simulink model "NavigationObserver_4"  (Simulink 8.3)
settings: configuration reference "mpc555rt_ref_debug_config" (kept outside this file)
values from neighbouring files (symbols this model uses):
  dt = 0.0192307692308    [newvars_4_25.mat]
  g = 32.174    [newvars_4_25.mat]
  P0_est_nav = [100 0 0 0 0 0 0 100 0 0 0 0 ... (36 elements, 6x6)]    [newvars_4_25.mat]
  Q_obs_nav = [0.001 0 0 0 0 0 0 0.001 0 0 0 0 ... (36 elements, 6x6)]    [newvars_4_25.mat]
  R_obs_nav = [0.001 0 0 0 0 0 0 0.001 0 0 0 0 ... (36 elements, 6x6)]    [newvars_4_25.mat]
  x0_est_nav = [0 0 200 0 0 0]    [newvars_4_25.mat]
libraries: simulink x1
(part 2 of 2)

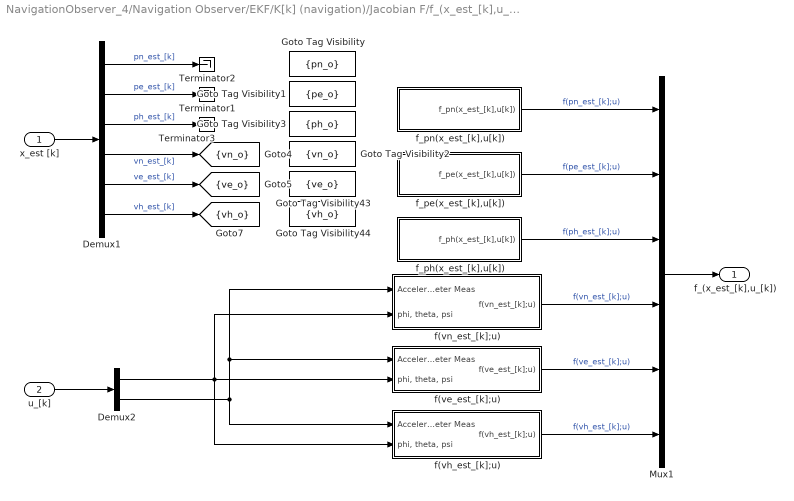
== system NavigationObserver_4/Navigation Observer/EKF/K[k] (navigation)/Jacobian F/f_(x_est_[k],u_[k])+delta_ve/f(x_est_[k],u_[k]) ==
  x_est [k] : Inport
  u_[k] : Inport  Port=2
  Demux1 : Demux  Outputs=6
  Demux2 : Demux  Outputs=2
  Goto Tag Visibility : GotoTagVisibility  GotoTag=pn_o
  Goto Tag Visibility1 : GotoTagVisibility  GotoTag=pe_o
  Goto Tag Visibility2 : GotoTagVisibility  GotoTag=vn_o
  Goto Tag Visibility3 : GotoTagVisibility  GotoTag=ph_o
  Goto Tag Visibility43 : GotoTagVisibility  GotoTag=ve_o
  Goto Tag Visibility44 : GotoTagVisibility  GotoTag=vh_o
  Mux1 : Mux  Inputs=6
  Terminator1 : Terminator
  Terminator2 : Terminator
  Terminator3 : Terminator
  f(ve_est_[k];u) : Subsystem
  f(vh_est_[k];u) : Subsystem
  f(vn_est_[k];u) : Subsystem
  f_pe(x_est_[k],u[k]) : Subsystem
  f_ph(x_est_[k],u[k]) : Subsystem
  f_pn(x_est_[k],u[k]) : Subsystem
  f_(x_est_[k],u_[k]) : Outport
  tag scope: ve_o=scoped, vh_o=scoped, vn_o=scoped
  wires:
  Demux2/2 -> f(vh_est_[k];u)/1(Accelerometer Meas), f(ve_est_[k];u)/1(Accelerometer Meas), f(vn_est_[k];u)/1(Accelerometer Meas)
  Demux2/1 -> f(vn_est_[k];u)/2("phi, theta, psi"), f(vh_est_[k];u)/2("phi, theta, psi"), f(ve_est_[k];u)/2("phi, theta, psi")
  u_[k]/1 -> Demux2/1
  f_pe(x_est_[k],u[k])/1(f_pe(x_est_[k],u[k])) -> Mux1/2  "f(pe_est_[k];u)"
  f_pn(x_est_[k],u[k])/1(f_pn(x_est_[k],u[k])) -> Mux1/1  "f(pn_est_[k];u)"
  f_ph(x_est_[k],u[k])/1(f_ph(x_est_[k],u[k])) -> Mux1/3  "f(ph_est_[k];u)"
  f(vn_est_[k];u)/1(f(vn_est_[k];u)) -> Mux1/4  "f(vn_est_[k];u)"
  f(ve_est_[k];u)/1(f(ve_est_[k];u)) -> Mux1/5  "f(ve_est_[k];u)"
  Mux1/1 -> f_(x_est_[k],u_[k])/1
  f(vh_est_[k];u)/1(f(vh_est_[k];u)) -> Mux1/6  "f(vh_est_[k];u)"
  Demux1/5 -> [ve_o]  "ve_est_[k]"
  x_est [k]/1 -> Demux1/1
  Demux1/6 -> [vh_o]  "vh_est_[k]"
  Demux1/4 -> [vn_o]  "vn_est_[k]"
  Demux1/3 -> Terminator3/1  "ph_est_[k]"
  Demux1/2 -> Terminator1/1  "pe_est_[k]"
  Demux1/1 -> Terminator2/1  "pn_est_[k]"

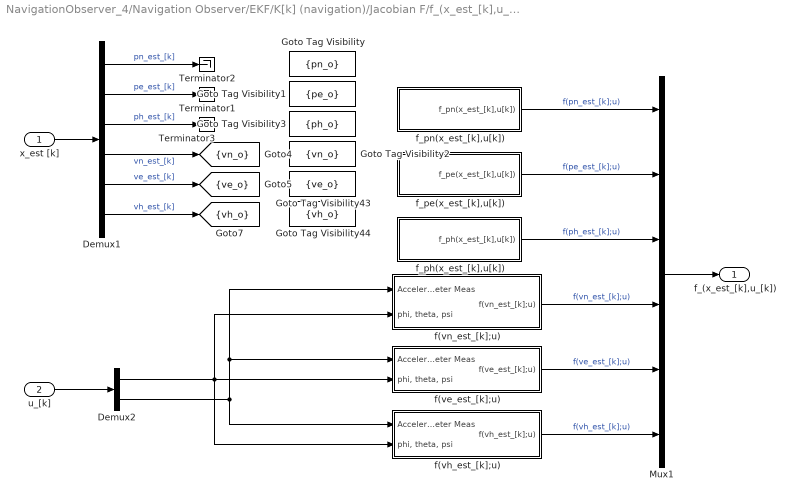
== system NavigationObserver_4/Navigation Observer/EKF/K[k] (navigation)/Jacobian F/f_(x_est_[k],u_[k])+delta_vh/f(x_est_[k],u_[k]) ==
  x_est [k] : Inport
  u_[k] : Inport  Port=2
  Demux1 : Demux  Outputs=6
  Demux2 : Demux  Outputs=2
  Goto Tag Visibility : GotoTagVisibility  GotoTag=pn_o
  Goto Tag Visibility1 : GotoTagVisibility  GotoTag=pe_o
  Goto Tag Visibility2 : GotoTagVisibility  GotoTag=vn_o
  Goto Tag Visibility3 : GotoTagVisibility  GotoTag=ph_o
  Goto Tag Visibility43 : GotoTagVisibility  GotoTag=ve_o
  Goto Tag Visibility44 : GotoTagVisibility  GotoTag=vh_o
  Mux1 : Mux  Inputs=6
  Terminator1 : Terminator
  Terminator2 : Terminator
  Terminator3 : Terminator
  f(ve_est_[k];u) : Subsystem
  f(vh_est_[k];u) : Subsystem
  f(vn_est_[k];u) : Subsystem
  f_pe(x_est_[k],u[k]) : Subsystem
  f_ph(x_est_[k],u[k]) : Subsystem
  f_pn(x_est_[k],u[k]) : Subsystem
  f_(x_est_[k],u_[k]) : Outport
  tag scope: ve_o=scoped, vh_o=scoped, vn_o=scoped
  wires:
  Demux2/2 -> f(vh_est_[k];u)/1(Accelerometer Meas), f(ve_est_[k];u)/1(Accelerometer Meas), f(vn_est_[k];u)/1(Accelerometer Meas)
  Demux2/1 -> f(vn_est_[k];u)/2("phi, theta, psi"), f(vh_est_[k];u)/2("phi, theta, psi"), f(ve_est_[k];u)/2("phi, theta, psi")
  u_[k]/1 -> Demux2/1
  f_pe(x_est_[k],u[k])/1(f_pe(x_est_[k],u[k])) -> Mux1/2  "f(pe_est_[k];u)"
  f_pn(x_est_[k],u[k])/1(f_pn(x_est_[k],u[k])) -> Mux1/1  "f(pn_est_[k];u)"
  f_ph(x_est_[k],u[k])/1(f_ph(x_est_[k],u[k])) -> Mux1/3  "f(ph_est_[k];u)"
  f(vn_est_[k];u)/1(f(vn_est_[k];u)) -> Mux1/4  "f(vn_est_[k];u)"
  f(ve_est_[k];u)/1(f(ve_est_[k];u)) -> Mux1/5  "f(ve_est_[k];u)"
  Mux1/1 -> f_(x_est_[k],u_[k])/1
  f(vh_est_[k];u)/1(f(vh_est_[k];u)) -> Mux1/6  "f(vh_est_[k];u)"
  Demux1/5 -> [ve_o]  "ve_est_[k]"
  x_est [k]/1 -> Demux1/1
  Demux1/6 -> [vh_o]  "vh_est_[k]"
  Demux1/4 -> [vn_o]  "vn_est_[k]"
  Demux1/3 -> Terminator3/1  "ph_est_[k]"
  Demux1/2 -> Terminator1/1  "pe_est_[k]"
  Demux1/1 -> Terminator2/1  "pn_est_[k]"

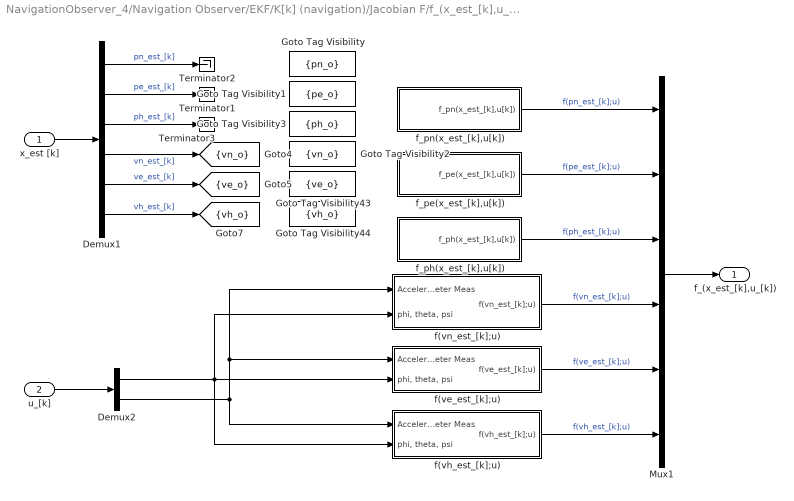
== system NavigationObserver_4/Navigation Observer/EKF/K[k] (navigation)/Jacobian F/f_(x_est_[k],u_[k])+delta_vn/f(x_est_[k],u_[k]) ==
  x_est [k] : Inport
  u_[k] : Inport  Port=2
  Demux1 : Demux  Outputs=6
  Demux2 : Demux  Outputs=2
  Goto Tag Visibility : GotoTagVisibility  GotoTag=pn_o
  Goto Tag Visibility1 : GotoTagVisibility  GotoTag=pe_o
  Goto Tag Visibility2 : GotoTagVisibility  GotoTag=vn_o
  Goto Tag Visibility3 : GotoTagVisibility  GotoTag=ph_o
  Goto Tag Visibility43 : GotoTagVisibility  GotoTag=ve_o
  Goto Tag Visibility44 : GotoTagVisibility  GotoTag=vh_o
  Mux1 : Mux  Inputs=6
  Terminator1 : Terminator
  Terminator2 : Terminator
  Terminator3 : Terminator
  f(ve_est_[k];u) : Subsystem
  f(vh_est_[k];u) : Subsystem
  f(vn_est_[k];u) : Subsystem
  f_pe(x_est_[k],u[k]) : Subsystem
  f_ph(x_est_[k],u[k]) : Subsystem
  f_pn(x_est_[k],u[k]) : Subsystem
  f_(x_est_[k],u_[k]) : Outport
  tag scope: ve_o=scoped, vh_o=scoped, vn_o=scoped
  wires:
  Demux2/2 -> f(vh_est_[k];u)/1(Accelerometer Meas), f(ve_est_[k];u)/1(Accelerometer Meas), f(vn_est_[k];u)/1(Accelerometer Meas)
  Demux2/1 -> f(vn_est_[k];u)/2("phi, theta, psi"), f(vh_est_[k];u)/2("phi, theta, psi"), f(ve_est_[k];u)/2("phi, theta, psi")
  u_[k]/1 -> Demux2/1
  f_pe(x_est_[k],u[k])/1(f_pe(x_est_[k],u[k])) -> Mux1/2  "f(pe_est_[k];u)"
  f_pn(x_est_[k],u[k])/1(f_pn(x_est_[k],u[k])) -> Mux1/1  "f(pn_est_[k];u)"
  f_ph(x_est_[k],u[k])/1(f_ph(x_est_[k],u[k])) -> Mux1/3  "f(ph_est_[k];u)"
  f(vn_est_[k];u)/1(f(vn_est_[k];u)) -> Mux1/4  "f(vn_est_[k];u)"
  f(ve_est_[k];u)/1(f(ve_est_[k];u)) -> Mux1/5  "f(ve_est_[k];u)"
  Mux1/1 -> f_(x_est_[k],u_[k])/1
  f(vh_est_[k];u)/1(f(vh_est_[k];u)) -> Mux1/6  "f(vh_est_[k];u)"
  Demux1/5 -> [ve_o]  "ve_est_[k]"
  x_est [k]/1 -> Demux1/1
  Demux1/6 -> [vh_o]  "vh_est_[k]"
  Demux1/4 -> [vn_o]  "vn_est_[k]"
  Demux1/3 -> Terminator3/1  "ph_est_[k]"
  Demux1/2 -> Terminator1/1  "pe_est_[k]"
  Demux1/1 -> Terminator2/1  "pn_est_[k]"

== system NavigationObserver_4/Navigation Observer/EKF/K[k] (navigation)/Jacobian F/f_(x_est_[k],u_[k])/f(x_est_[k],u_[k])/f(ve_est_[k];u) ==
  note: psi [rad]
  note: phi [rad]
  note: theta [rad]
  note: az [ft/sec2]
  note: ay [ft/sec2]
  note: ax [ft/sec2]
  Accelerometer Meas : Inport
  "phi, theta, psi" : Inport  Port=2
  Add1 : Sum
  Add2 : Sum  Inputs=+++
  Add3 : Sum  Inputs=-+
  Demux1 : Demux  Outputs=3
  Demux2 : Demux  Outputs=3
  Divide{1,4,6..7} (4 alike) : Product  Inputs=**
  Divide2 : Product  Inputs=***
  Divide3 : Product  Inputs=***
  Divide5 : Product  Inputs=***
  Trigonometric Function : Trigonometry
  Trigonometric Function1 : Trigonometry  Operator=cos
  Trigonometric Function2 : Trigonometry
  Trigonometric Function3 : Trigonometry
  Trigonometric Function4 : Trigonometry  Operator=cos
  Trigonometric Function5 : Trigonometry  Operator=cos
  f(ve_est_[k];u) : Outport
  wires:
  "phi, theta, psi"/1 -> Demux2/1
  Accelerometer Meas/1 -> Demux1/1
  Add2/1 -> f(ve_est_[k];u)/1
  Demux1/1 -> Divide3/1
  Trigonometric Function1/1 -> Divide3/2
  Add1/1 -> Divide1/1
  Divide4/1 -> Add1/1
  Divide2/1 -> Add1/2
  Divide3/1 -> Add2/1
  Divide1/1 -> Add2/2
  Divide6/1 -> Add3/1
  Divide5/1 -> Add3/2
  Add3/1 -> Divide7/1
  Divide7/1 -> Add2/3
  Trigonometric Function3/1 -> Divide2/3, Divide5/3, Divide3/3
  Trigonometric Function5/1 -> Divide4/1, Divide5/2
  Trigonometric Function4/1 -> Divide4/2, Divide6/2
  Trigonometric Function2/1 -> Divide2/1, Divide5/1
  Trigonometric Function/1 -> Divide2/2, Divide6/1
  Demux1/3 -> Divide7/2
  Demux1/2 -> Divide1/2
  Demux2/1 -> Trigonometric Function5/1, Trigonometric Function/1
  Demux2/2 -> Trigonometric Function1/1, Trigonometric Function2/1
  Demux2/3 -> Trigonometric Function4/1, Trigonometric Function3/1

== system NavigationObserver_4/Navigation Observer/EKF/K[k] (navigation)/Jacobian F/f_(x_est_[k],u_[k])/f(x_est_[k],u_[k])/f(vh_est_[k];u) ==
  note: phi [rad]
  note: theta [rad]
  note: az [ft/sec2]
  note: ay [ft/sec2]
  note: ax [ft/sec2]
  Accelerometer Meas : Inport
  "phi, theta, psi" : Inport  Port=2
  Add1 : Sum  Inputs=+--
  Demux1 : Demux  Outputs=3
  Demux2 : Demux  Outputs=3
  Divide1 : Product  Inputs=***
  Divide2 : Product  Inputs=**
  Divide3 : Product  Inputs=***
  Sum : Sum  Inputs=|+-  SampleTime=dt
  Terminator2 : Terminator
  Trigonometric Function : Trigonometry
  Trigonometric Function1 : Trigonometry  Operator=cos
  Trigonometric Function2 : Trigonometry
  Trigonometric Function4 : Trigonometry  Operator=cos
  Trigonometric Function5 : Trigonometry  Operator=cos
  gravity : Constant  Value=g
  f(vh_est_[k];u) : Outport
  wires:
  gravity/1 -> Sum/2
  Sum/1 -> f(vh_est_[k];u)/1
  Add1/1 -> Sum/1
  Demux2/3 -> Terminator2/1
  "phi, theta, psi"/1 -> Demux2/1
  Accelerometer Meas/1 -> Demux1/1
  Demux1/1 -> Divide2/1
  Trigonometric Function/1 -> Divide2/2
  Trigonometric Function1/1 -> Divide3/1
  Trigonometric Function2/1 -> Divide3/2
  Demux1/2 -> Divide3/3
  Divide3/1 -> Add1/2
  Divide2/1 -> Add1/1
  Trigonometric Function4/1 -> Divide1/1
  Trigonometric Function5/1 -> Divide1/2
  Demux1/3 -> Divide1/3
  Divide1/1 -> Add1/3
  Demux2/2 -> Trigonometric Function/1, Trigonometric Function1/1, Trigonometric Function5/1
  Demux2/1 -> Trigonometric Function2/1, Trigonometric Function4/1

== system NavigationObserver_4/Navigation Observer/EKF/K[k] (navigation)/Jacobian F/f_(x_est_[k],u_[k])/f(x_est_[k],u_[k])/f(vn_est_[k];u) ==
  note: psi [rad]
  note: phi [rad]
  note: theta [rad]
  note: az [ft/sec2]
  note: ay [ft/sec2]
  note: ax [ft/sec2]
  Accelerometer Meas : Inport
  "phi, theta, psi" : Inport  Port=2
  Add1 : Sum  Inputs=-+
  Add2 : Sum  Inputs=+++
  Add3 : Sum
  Demux1 : Demux  Outputs=3
  Demux2 : Demux  Outputs=3
  Divide{1,4,6..7} (4 alike) : Product  Inputs=**
  Divide2 : Product  Inputs=***
  Divide3 : Product  Inputs=***
  Divide5 : Product  Inputs=***
  Trigonometric Function : Trigonometry
  Trigonometric Function1 : Trigonometry  Operator=cos
  Trigonometric Function2 : Trigonometry
  Trigonometric Function3 : Trigonometry
  Trigonometric Function4 : Trigonometry  Operator=cos
  Trigonometric Function5 : Trigonometry  Operator=cos
  f(vn_est_[k];u) : Outport
  wires:
  Accelerometer Meas/1 -> Demux1/1
  Demux1/1 -> Divide3/1
  Demux1/2 -> Divide1/2
  Demux1/3 -> Divide7/2
  Add2/1 -> f(vn_est_[k];u)/1
  Demux2/2 -> Trigonometric Function1/1, Trigonometric Function2/1
  Demux2/1 -> Trigonometric Function5/1, Trigonometric Function/1
  Demux2/3 -> Trigonometric Function4/1, Trigonometric Function3/1
  Trigonometric Function1/1 -> Divide3/2
  Trigonometric Function4/1 -> Divide3/3, Divide2/3, Divide5/3
  Add1/1 -> Divide1/1
  Divide4/1 -> Add1/1
  Divide2/1 -> Add1/2
  Trigonometric Function5/1 -> Divide4/1, Divide5/2
  Trigonometric Function3/1 -> Divide4/2, Divide6/2
  Trigonometric Function2/1 -> Divide2/1, Divide5/1
  Trigonometric Function/1 -> Divide2/2, Divide6/1
  Divide3/1 -> Add2/1
  Divide1/1 -> Add2/2
  Divide6/1 -> Add3/1
  Divide5/1 -> Add3/2
  Add3/1 -> Divide7/1
  Divide7/1 -> Add2/3
  "phi, theta, psi"/1 -> Demux2/1

== system NavigationObserver_4/Navigation Observer/EKF/K[k] (navigation)/Jacobian F/f_(x_est_[k],u_[k])/f(x_est_[k],u_[k])/f_pe(x_est_[k],u[k]) ==
  Gain : Gain
  f_pe(x_est_[k],u[k]) : Outport
  wires:
  Gain/1 -> f_pe(x_est_[k],u[k])/1
  [ve_o] -> Gain/1

== system NavigationObserver_4/Navigation Observer/EKF/K[k] (navigation)/Jacobian F/f_(x_est_[k],u_[k])/f(x_est_[k],u_[k])/f_ph(x_est_[k],u[k]) ==
  Gain : Gain
  f_ph(x_est_[k],u[k]) : Outport
  wires:
  Gain/1 -> f_ph(x_est_[k],u[k])/1
  [vh_o] -> Gain/1

== system NavigationObserver_4/Navigation Observer/EKF/K[k] (navigation)/Jacobian F/f_(x_est_[k],u_[k])/f(x_est_[k],u_[k])/f_pn(x_est_[k],u[k]) ==
  Gain : Gain
  f_pn(x_est_[k],u[k]) : Outport
  wires:
  Gain/1 -> f_pn(x_est_[k],u[k])/1
  [vn_o] -> Gain/1

== system NavigationObserver_4/Navigation Observer/EKF/K[k] (navigation)/Jacobian F/f_(x_est_[k],u_[k])+delta_pe/f(x_est_[k],u_[k])/f(ve_est_[k];u) ==
  note: psi [rad]
  note: phi [rad]
  note: theta [rad]
  note: az [ft/sec2]
  note: ay [ft/sec2]
  note: ax [ft/sec2]
  Accelerometer Meas : Inport
  "phi, theta, psi" : Inport  Port=2
  Add1 : Sum
  Add2 : Sum  Inputs=+++
  Add3 : Sum  Inputs=-+
  Demux1 : Demux  Outputs=3
  Demux2 : Demux  Outputs=3
  Divide{1,4,6..7} (4 alike) : Product  Inputs=**
  Divide2 : Product  Inputs=***
  Divide3 : Product  Inputs=***
  Divide5 : Product  Inputs=***
  Trigonometric Function : Trigonometry
  Trigonometric Function1 : Trigonometry  Operator=cos
  Trigonometric Function2 : Trigonometry
  Trigonometric Function3 : Trigonometry
  Trigonometric Function4 : Trigonometry  Operator=cos
  Trigonometric Function5 : Trigonometry  Operator=cos
  f(ve_est_[k];u) : Outport
  wires:
  "phi, theta, psi"/1 -> Demux2/1
  Accelerometer Meas/1 -> Demux1/1
  Add2/1 -> f(ve_est_[k];u)/1
  Demux1/1 -> Divide3/1
  Trigonometric Function1/1 -> Divide3/2
  Add1/1 -> Divide1/1
  Divide4/1 -> Add1/1
  Divide2/1 -> Add1/2
  Divide3/1 -> Add2/1
  Divide1/1 -> Add2/2
  Divide6/1 -> Add3/1
  Divide5/1 -> Add3/2
  Add3/1 -> Divide7/1
  Divide7/1 -> Add2/3
  Trigonometric Function3/1 -> Divide2/3, Divide5/3, Divide3/3
  Trigonometric Function5/1 -> Divide4/1, Divide5/2
  Trigonometric Function4/1 -> Divide4/2, Divide6/2
  Trigonometric Function2/1 -> Divide2/1, Divide5/1
  Trigonometric Function/1 -> Divide2/2, Divide6/1
  Demux1/3 -> Divide7/2
  Demux1/2 -> Divide1/2
  Demux2/1 -> Trigonometric Function5/1, Trigonometric Function/1
  Demux2/2 -> Trigonometric Function1/1, Trigonometric Function2/1
  Demux2/3 -> Trigonometric Function4/1, Trigonometric Function3/1

== system NavigationObserver_4/Navigation Observer/EKF/K[k] (navigation)/Jacobian F/f_(x_est_[k],u_[k])+delta_pe/f(x_est_[k],u_[k])/f(vh_est_[k];u) ==
  note: phi [rad]
  note: theta [rad]
  note: az [ft/sec2]
  note: ay [ft/sec2]
  note: ax [ft/sec2]
  Accelerometer Meas : Inport
  "phi, theta, psi" : Inport  Port=2
  Add1 : Sum  Inputs=+--
  Demux1 : Demux  Outputs=3
  Demux2 : Demux  Outputs=3
  Divide1 : Product  Inputs=***
  Divide2 : Product  Inputs=**
  Divide3 : Product  Inputs=***
  Sum : Sum  Inputs=|+-  SampleTime=dt
  Terminator2 : Terminator
  Trigonometric Function : Trigonometry
  Trigonometric Function1 : Trigonometry  Operator=cos
  Trigonometric Function2 : Trigonometry
  Trigonometric Function4 : Trigonometry  Operator=cos
  Trigonometric Function5 : Trigonometry  Operator=cos
  gravity : Constant  Value=g
  f(vh_est_[k];u) : Outport
  wires:
  gravity/1 -> Sum/2
  Sum/1 -> f(vh_est_[k];u)/1
  Add1/1 -> Sum/1
  Demux2/3 -> Terminator2/1
  "phi, theta, psi"/1 -> Demux2/1
  Accelerometer Meas/1 -> Demux1/1
  Demux1/1 -> Divide2/1
  Trigonometric Function/1 -> Divide2/2
  Trigonometric Function1/1 -> Divide3/1
  Trigonometric Function2/1 -> Divide3/2
  Demux1/2 -> Divide3/3
  Divide3/1 -> Add1/2
  Divide2/1 -> Add1/1
  Trigonometric Function4/1 -> Divide1/1
  Trigonometric Function5/1 -> Divide1/2
  Demux1/3 -> Divide1/3
  Divide1/1 -> Add1/3
  Demux2/2 -> Trigonometric Function/1, Trigonometric Function1/1, Trigonometric Function5/1
  Demux2/1 -> Trigonometric Function2/1, Trigonometric Function4/1

== system NavigationObserver_4/Navigation Observer/EKF/K[k] (navigation)/Jacobian F/f_(x_est_[k],u_[k])+delta_pe/f(x_est_[k],u_[k])/f(vn_est_[k];u) ==
  note: psi [rad]
  note: phi [rad]
  note: theta [rad]
  note: az [ft/sec2]
  note: ay [ft/sec2]
  note: ax [ft/sec2]
  Accelerometer Meas : Inport
  "phi, theta, psi" : Inport  Port=2
  Add1 : Sum  Inputs=-+
  Add2 : Sum  Inputs=+++
  Add3 : Sum
  Demux1 : Demux  Outputs=3
  Demux2 : Demux  Outputs=3
  Divide{1,4,6..7} (4 alike) : Product  Inputs=**
  Divide2 : Product  Inputs=***
  Divide3 : Product  Inputs=***
  Divide5 : Product  Inputs=***
  Trigonometric Function : Trigonometry
  Trigonometric Function1 : Trigonometry  Operator=cos
  Trigonometric Function2 : Trigonometry
  Trigonometric Function3 : Trigonometry
  Trigonometric Function4 : Trigonometry  Operator=cos
  Trigonometric Function5 : Trigonometry  Operator=cos
  f(vn_est_[k];u) : Outport
  wires:
  Accelerometer Meas/1 -> Demux1/1
  Demux1/1 -> Divide3/1
  Demux1/2 -> Divide1/2
  Demux1/3 -> Divide7/2
  Add2/1 -> f(vn_est_[k];u)/1
  Demux2/2 -> Trigonometric Function1/1, Trigonometric Function2/1
  Demux2/1 -> Trigonometric Function5/1, Trigonometric Function/1
  Demux2/3 -> Trigonometric Function4/1, Trigonometric Function3/1
  Trigonometric Function1/1 -> Divide3/2
  Trigonometric Function4/1 -> Divide3/3, Divide2/3, Divide5/3
  Add1/1 -> Divide1/1
  Divide4/1 -> Add1/1
  Divide2/1 -> Add1/2
  Trigonometric Function5/1 -> Divide4/1, Divide5/2
  Trigonometric Function3/1 -> Divide4/2, Divide6/2
  Trigonometric Function2/1 -> Divide2/1, Divide5/1
  Trigonometric Function/1 -> Divide2/2, Divide6/1
  Divide3/1 -> Add2/1
  Divide1/1 -> Add2/2
  Divide6/1 -> Add3/1
  Divide5/1 -> Add3/2
  Add3/1 -> Divide7/1
  Divide7/1 -> Add2/3
  "phi, theta, psi"/1 -> Demux2/1

== system NavigationObserver_4/Navigation Observer/EKF/K[k] (navigation)/Jacobian F/f_(x_est_[k],u_[k])+delta_pe/f(x_est_[k],u_[k])/f_pe(x_est_[k],u[k]) ==
  Gain : Gain
  f_pe(x_est_[k],u[k]) : Outport
  wires:
  Gain/1 -> f_pe(x_est_[k],u[k])/1
  [ve_o] -> Gain/1

== system NavigationObserver_4/Navigation Observer/EKF/K[k] (navigation)/Jacobian F/f_(x_est_[k],u_[k])+delta_pe/f(x_est_[k],u_[k])/f_ph(x_est_[k],u[k]) ==
  Gain : Gain
  f_ph(x_est_[k],u[k]) : Outport
  wires:
  Gain/1 -> f_ph(x_est_[k],u[k])/1
  [vh_o] -> Gain/1

== system NavigationObserver_4/Navigation Observer/EKF/K[k] (navigation)/Jacobian F/f_(x_est_[k],u_[k])+delta_pe/f(x_est_[k],u_[k])/f_pn(x_est_[k],u[k]) ==
  Gain : Gain
  f_pn(x_est_[k],u[k]) : Outport
  wires:
  Gain/1 -> f_pn(x_est_[k],u[k])/1
  [vn_o] -> Gain/1

== system NavigationObserver_4/Navigation Observer/EKF/K[k] (navigation)/Jacobian F/f_(x_est_[k],u_[k])+delta_ph/f(x_est_[k],u_[k])/f(ve_est_[k];u) ==
  note: psi [rad]
  note: phi [rad]
  note: theta [rad]
  note: az [ft/sec2]
  note: ay [ft/sec2]
  note: ax [ft/sec2]
  Accelerometer Meas : Inport
  "phi, theta, psi" : Inport  Port=2
  Add1 : Sum
  Add2 : Sum  Inputs=+++
  Add3 : Sum  Inputs=-+
  Demux1 : Demux  Outputs=3
  Demux2 : Demux  Outputs=3
  Divide{1,4,6..7} (4 alike) : Product  Inputs=**
  Divide2 : Product  Inputs=***
  Divide3 : Product  Inputs=***
  Divide5 : Product  Inputs=***
  Trigonometric Function : Trigonometry
  Trigonometric Function1 : Trigonometry  Operator=cos
  Trigonometric Function2 : Trigonometry
  Trigonometric Function3 : Trigonometry
  Trigonometric Function4 : Trigonometry  Operator=cos
  Trigonometric Function5 : Trigonometry  Operator=cos
  f(ve_est_[k];u) : Outport
  wires:
  "phi, theta, psi"/1 -> Demux2/1
  Accelerometer Meas/1 -> Demux1/1
  Add2/1 -> f(ve_est_[k];u)/1
  Demux1/1 -> Divide3/1
  Trigonometric Function1/1 -> Divide3/2
  Add1/1 -> Divide1/1
  Divide4/1 -> Add1/1
  Divide2/1 -> Add1/2
  Divide3/1 -> Add2/1
  Divide1/1 -> Add2/2
  Divide6/1 -> Add3/1
  Divide5/1 -> Add3/2
  Add3/1 -> Divide7/1
  Divide7/1 -> Add2/3
  Trigonometric Function3/1 -> Divide2/3, Divide5/3, Divide3/3
  Trigonometric Function5/1 -> Divide4/1, Divide5/2
  Trigonometric Function4/1 -> Divide4/2, Divide6/2
  Trigonometric Function2/1 -> Divide2/1, Divide5/1
  Trigonometric Function/1 -> Divide2/2, Divide6/1
  Demux1/3 -> Divide7/2
  Demux1/2 -> Divide1/2
  Demux2/1 -> Trigonometric Function5/1, Trigonometric Function/1
  Demux2/2 -> Trigonometric Function1/1, Trigonometric Function2/1
  Demux2/3 -> Trigonometric Function4/1, Trigonometric Function3/1

== system NavigationObserver_4/Navigation Observer/EKF/K[k] (navigation)/Jacobian F/f_(x_est_[k],u_[k])+delta_ph/f(x_est_[k],u_[k])/f(vh_est_[k];u) ==
  note: phi [rad]
  note: theta [rad]
  note: az [ft/sec2]
  note: ay [ft/sec2]
  note: ax [ft/sec2]
  Accelerometer Meas : Inport
  "phi, theta, psi" : Inport  Port=2
  Add1 : Sum  Inputs=+--
  Demux1 : Demux  Outputs=3
  Demux2 : Demux  Outputs=3
  Divide1 : Product  Inputs=***
  Divide2 : Product  Inputs=**
  Divide3 : Product  Inputs=***
  Sum : Sum  Inputs=|+-  SampleTime=dt
  Terminator2 : Terminator
  Trigonometric Function : Trigonometry
  Trigonometric Function1 : Trigonometry  Operator=cos
  Trigonometric Function2 : Trigonometry
  Trigonometric Function4 : Trigonometry  Operator=cos
  Trigonometric Function5 : Trigonometry  Operator=cos
  gravity : Constant  Value=g
  f(vh_est_[k];u) : Outport
  wires:
  gravity/1 -> Sum/2
  Sum/1 -> f(vh_est_[k];u)/1
  Add1/1 -> Sum/1
  Demux2/3 -> Terminator2/1
  "phi, theta, psi"/1 -> Demux2/1
  Accelerometer Meas/1 -> Demux1/1
  Demux1/1 -> Divide2/1
  Trigonometric Function/1 -> Divide2/2
  Trigonometric Function1/1 -> Divide3/1
  Trigonometric Function2/1 -> Divide3/2
  Demux1/2 -> Divide3/3
  Divide3/1 -> Add1/2
  Divide2/1 -> Add1/1
  Trigonometric Function4/1 -> Divide1/1
  Trigonometric Function5/1 -> Divide1/2
  Demux1/3 -> Divide1/3
  Divide1/1 -> Add1/3
  Demux2/2 -> Trigonometric Function/1, Trigonometric Function1/1, Trigonometric Function5/1
  Demux2/1 -> Trigonometric Function2/1, Trigonometric Function4/1

== system NavigationObserver_4/Navigation Observer/EKF/K[k] (navigation)/Jacobian F/f_(x_est_[k],u_[k])+delta_ph/f(x_est_[k],u_[k])/f(vn_est_[k];u) ==
  note: psi [rad]
  note: phi [rad]
  note: theta [rad]
  note: az [ft/sec2]
  note: ay [ft/sec2]
  note: ax [ft/sec2]
  Accelerometer Meas : Inport
  "phi, theta, psi" : Inport  Port=2
  Add1 : Sum  Inputs=-+
  Add2 : Sum  Inputs=+++
  Add3 : Sum
  Demux1 : Demux  Outputs=3
  Demux2 : Demux  Outputs=3
  Divide{1,4,6..7} (4 alike) : Product  Inputs=**
  Divide2 : Product  Inputs=***
  Divide3 : Product  Inputs=***
  Divide5 : Product  Inputs=***
  Trigonometric Function : Trigonometry
  Trigonometric Function1 : Trigonometry  Operator=cos
  Trigonometric Function2 : Trigonometry
  Trigonometric Function3 : Trigonometry
  Trigonometric Function4 : Trigonometry  Operator=cos
  Trigonometric Function5 : Trigonometry  Operator=cos
  f(vn_est_[k];u) : Outport
  wires:
  Accelerometer Meas/1 -> Demux1/1
  Demux1/1 -> Divide3/1
  Demux1/2 -> Divide1/2
  Demux1/3 -> Divide7/2
  Add2/1 -> f(vn_est_[k];u)/1
  Demux2/2 -> Trigonometric Function1/1, Trigonometric Function2/1
  Demux2/1 -> Trigonometric Function5/1, Trigonometric Function/1
  Demux2/3 -> Trigonometric Function4/1, Trigonometric Function3/1
  Trigonometric Function1/1 -> Divide3/2
  Trigonometric Function4/1 -> Divide3/3, Divide2/3, Divide5/3
  Add1/1 -> Divide1/1
  Divide4/1 -> Add1/1
  Divide2/1 -> Add1/2
  Trigonometric Function5/1 -> Divide4/1, Divide5/2
  Trigonometric Function3/1 -> Divide4/2, Divide6/2
  Trigonometric Function2/1 -> Divide2/1, Divide5/1
  Trigonometric Function/1 -> Divide2/2, Divide6/1
  Divide3/1 -> Add2/1
  Divide1/1 -> Add2/2
  Divide6/1 -> Add3/1
  Divide5/1 -> Add3/2
  Add3/1 -> Divide7/1
  Divide7/1 -> Add2/3
  "phi, theta, psi"/1 -> Demux2/1

== system NavigationObserver_4/Navigation Observer/EKF/K[k] (navigation)/Jacobian F/f_(x_est_[k],u_[k])+delta_ph/f(x_est_[k],u_[k])/f_pe(x_est_[k],u[k]) ==
  Gain : Gain
  f_pe(x_est_[k],u[k]) : Outport
  wires:
  Gain/1 -> f_pe(x_est_[k],u[k])/1
  [ve_o] -> Gain/1

== system NavigationObserver_4/Navigation Observer/EKF/K[k] (navigation)/Jacobian F/f_(x_est_[k],u_[k])+delta_ph/f(x_est_[k],u_[k])/f_ph(x_est_[k],u[k]) ==
  Gain : Gain
  f_ph(x_est_[k],u[k]) : Outport
  wires:
  Gain/1 -> f_ph(x_est_[k],u[k])/1
  [vh_o] -> Gain/1

== system NavigationObserver_4/Navigation Observer/EKF/K[k] (navigation)/Jacobian F/f_(x_est_[k],u_[k])+delta_ph/f(x_est_[k],u_[k])/f_pn(x_est_[k],u[k]) ==
  Gain : Gain
  f_pn(x_est_[k],u[k]) : Outport
  wires:
  Gain/1 -> f_pn(x_est_[k],u[k])/1
  [vn_o] -> Gain/1

== system NavigationObserver_4/Navigation Observer/EKF/K[k] (navigation)/Jacobian F/f_(x_est_[k],u_[k])+delta_pn/f(x_est_[k],u_[k])/f(ve_est_[k];u) ==
  note: psi [rad]
  note: phi [rad]
  note: theta [rad]
  note: az [ft/sec2]
  note: ay [ft/sec2]
  note: ax [ft/sec2]
  Accelerometer Meas : Inport
  "phi, theta, psi" : Inport  Port=2
  Add1 : Sum
  Add2 : Sum  Inputs=+++
  Add3 : Sum  Inputs=-+
  Demux1 : Demux  Outputs=3
  Demux2 : Demux  Outputs=3
  Divide{1,4,6..7} (4 alike) : Product  Inputs=**
  Divide2 : Product  Inputs=***
  Divide3 : Product  Inputs=***
  Divide5 : Product  Inputs=***
  Trigonometric Function : Trigonometry
  Trigonometric Function1 : Trigonometry  Operator=cos
  Trigonometric Function2 : Trigonometry
  Trigonometric Function3 : Trigonometry
  Trigonometric Function4 : Trigonometry  Operator=cos
  Trigonometric Function5 : Trigonometry  Operator=cos
  f(ve_est_[k];u) : Outport
  wires:
  "phi, theta, psi"/1 -> Demux2/1
  Accelerometer Meas/1 -> Demux1/1
  Add2/1 -> f(ve_est_[k];u)/1
  Demux1/1 -> Divide3/1
  Trigonometric Function1/1 -> Divide3/2
  Add1/1 -> Divide1/1
  Divide4/1 -> Add1/1
  Divide2/1 -> Add1/2
  Divide3/1 -> Add2/1
  Divide1/1 -> Add2/2
  Divide6/1 -> Add3/1
  Divide5/1 -> Add3/2
  Add3/1 -> Divide7/1
  Divide7/1 -> Add2/3
  Trigonometric Function3/1 -> Divide2/3, Divide5/3, Divide3/3
  Trigonometric Function5/1 -> Divide4/1, Divide5/2
  Trigonometric Function4/1 -> Divide4/2, Divide6/2
  Trigonometric Function2/1 -> Divide2/1, Divide5/1
  Trigonometric Function/1 -> Divide2/2, Divide6/1
  Demux1/3 -> Divide7/2
  Demux1/2 -> Divide1/2
  Demux2/1 -> Trigonometric Function5/1, Trigonometric Function/1
  Demux2/2 -> Trigonometric Function1/1, Trigonometric Function2/1
  Demux2/3 -> Trigonometric Function4/1, Trigonometric Function3/1

== system NavigationObserver_4/Navigation Observer/EKF/K[k] (navigation)/Jacobian F/f_(x_est_[k],u_[k])+delta_pn/f(x_est_[k],u_[k])/f(vh_est_[k];u) ==
  note: phi [rad]
  note: theta [rad]
  note: az [ft/sec2]
  note: ay [ft/sec2]
  note: ax [ft/sec2]
  Accelerometer Meas : Inport
  "phi, theta, psi" : Inport  Port=2
  Add1 : Sum  Inputs=+--
  Demux1 : Demux  Outputs=3
  Demux2 : Demux  Outputs=3
  Divide1 : Product  Inputs=***
  Divide2 : Product  Inputs=**
  Divide3 : Product  Inputs=***
  Sum : Sum  Inputs=|+-  SampleTime=dt
  Terminator2 : Terminator
  Trigonometric Function : Trigonometry
  Trigonometric Function1 : Trigonometry  Operator=cos
  Trigonometric Function2 : Trigonometry
  Trigonometric Function4 : Trigonometry  Operator=cos
  Trigonometric Function5 : Trigonometry  Operator=cos
  gravity : Constant  Value=g
  f(vh_est_[k];u) : Outport
  wires:
  gravity/1 -> Sum/2
  Sum/1 -> f(vh_est_[k];u)/1
  Add1/1 -> Sum/1
  Demux2/3 -> Terminator2/1
  "phi, theta, psi"/1 -> Demux2/1
  Accelerometer Meas/1 -> Demux1/1
  Demux1/1 -> Divide2/1
  Trigonometric Function/1 -> Divide2/2
  Trigonometric Function1/1 -> Divide3/1
  Trigonometric Function2/1 -> Divide3/2
  Demux1/2 -> Divide3/3
  Divide3/1 -> Add1/2
  Divide2/1 -> Add1/1
  Trigonometric Function4/1 -> Divide1/1
  Trigonometric Function5/1 -> Divide1/2
  Demux1/3 -> Divide1/3
  Divide1/1 -> Add1/3
  Demux2/2 -> Trigonometric Function/1, Trigonometric Function1/1, Trigonometric Function5/1
  Demux2/1 -> Trigonometric Function2/1, Trigonometric Function4/1

== system NavigationObserver_4/Navigation Observer/EKF/K[k] (navigation)/Jacobian F/f_(x_est_[k],u_[k])+delta_pn/f(x_est_[k],u_[k])/f(vn_est_[k];u) ==
  note: psi [rad]
  note: phi [rad]
  note: theta [rad]
  note: az [ft/sec2]
  note: ay [ft/sec2]
  note: ax [ft/sec2]
  Accelerometer Meas : Inport
  "phi, theta, psi" : Inport  Port=2
  Add1 : Sum  Inputs=-+
  Add2 : Sum  Inputs=+++
  Add3 : Sum
  Demux1 : Demux  Outputs=3
  Demux2 : Demux  Outputs=3
  Divide{1,4,6..7} (4 alike) : Product  Inputs=**
  Divide2 : Product  Inputs=***
  Divide3 : Product  Inputs=***
  Divide5 : Product  Inputs=***
  Trigonometric Function : Trigonometry
  Trigonometric Function1 : Trigonometry  Operator=cos
  Trigonometric Function2 : Trigonometry
  Trigonometric Function3 : Trigonometry
  Trigonometric Function4 : Trigonometry  Operator=cos
  Trigonometric Function5 : Trigonometry  Operator=cos
  f(vn_est_[k];u) : Outport
  wires:
  Accelerometer Meas/1 -> Demux1/1
  Demux1/1 -> Divide3/1
  Demux1/2 -> Divide1/2
  Demux1/3 -> Divide7/2
  Add2/1 -> f(vn_est_[k];u)/1
  Demux2/2 -> Trigonometric Function1/1, Trigonometric Function2/1
  Demux2/1 -> Trigonometric Function5/1, Trigonometric Function/1
  Demux2/3 -> Trigonometric Function4/1, Trigonometric Function3/1
  Trigonometric Function1/1 -> Divide3/2
  Trigonometric Function4/1 -> Divide3/3, Divide2/3, Divide5/3
  Add1/1 -> Divide1/1
  Divide4/1 -> Add1/1
  Divide2/1 -> Add1/2
  Trigonometric Function5/1 -> Divide4/1, Divide5/2
  Trigonometric Function3/1 -> Divide4/2, Divide6/2
  Trigonometric Function2/1 -> Divide2/1, Divide5/1
  Trigonometric Function/1 -> Divide2/2, Divide6/1
  Divide3/1 -> Add2/1
  Divide1/1 -> Add2/2
  Divide6/1 -> Add3/1
  Divide5/1 -> Add3/2
  Add3/1 -> Divide7/1
  Divide7/1 -> Add2/3
  "phi, theta, psi"/1 -> Demux2/1

== system NavigationObserver_4/Navigation Observer/EKF/K[k] (navigation)/Jacobian F/f_(x_est_[k],u_[k])+delta_pn/f(x_est_[k],u_[k])/f_pe(x_est_[k],u[k]) ==
  Gain : Gain
  f_pe(x_est_[k],u[k]) : Outport
  wires:
  Gain/1 -> f_pe(x_est_[k],u[k])/1
  [ve_o] -> Gain/1

== system NavigationObserver_4/Navigation Observer/EKF/K[k] (navigation)/Jacobian F/f_(x_est_[k],u_[k])+delta_pn/f(x_est_[k],u_[k])/f_ph(x_est_[k],u[k]) ==
  Gain : Gain
  f_ph(x_est_[k],u[k]) : Outport
  wires:
  Gain/1 -> f_ph(x_est_[k],u[k])/1
  [vh_o] -> Gain/1

== system NavigationObserver_4/Navigation Observer/EKF/K[k] (navigation)/Jacobian F/f_(x_est_[k],u_[k])+delta_pn/f(x_est_[k],u_[k])/f_pn(x_est_[k],u[k]) ==
  Gain : Gain
  f_pn(x_est_[k],u[k]) : Outport
  wires:
  Gain/1 -> f_pn(x_est_[k],u[k])/1
  [vn_o] -> Gain/1

== system NavigationObserver_4/Navigation Observer/EKF/K[k] (navigation)/Jacobian F/f_(x_est_[k],u_[k])+delta_ve/f(x_est_[k],u_[k])/f(ve_est_[k];u) ==
  note: psi [rad]
  note: phi [rad]
  note: theta [rad]
  note: az [ft/sec2]
  note: ay [ft/sec2]
  note: ax [ft/sec2]
  Accelerometer Meas : Inport
  "phi, theta, psi" : Inport  Port=2
  Add1 : Sum
  Add2 : Sum  Inputs=+++
  Add3 : Sum  Inputs=-+
  Demux1 : Demux  Outputs=3
  Demux2 : Demux  Outputs=3
  Divide{1,4,6..7} (4 alike) : Product  Inputs=**
  Divide2 : Product  Inputs=***
  Divide3 : Product  Inputs=***
  Divide5 : Product  Inputs=***
  Trigonometric Function : Trigonometry
  Trigonometric Function1 : Trigonometry  Operator=cos
  Trigonometric Function2 : Trigonometry
  Trigonometric Function3 : Trigonometry
  Trigonometric Function4 : Trigonometry  Operator=cos
  Trigonometric Function5 : Trigonometry  Operator=cos
  f(ve_est_[k];u) : Outport
  wires:
  "phi, theta, psi"/1 -> Demux2/1
  Accelerometer Meas/1 -> Demux1/1
  Add2/1 -> f(ve_est_[k];u)/1
  Demux1/1 -> Divide3/1
  Trigonometric Function1/1 -> Divide3/2
  Add1/1 -> Divide1/1
  Divide4/1 -> Add1/1
  Divide2/1 -> Add1/2
  Divide3/1 -> Add2/1
  Divide1/1 -> Add2/2
  Divide6/1 -> Add3/1
  Divide5/1 -> Add3/2
  Add3/1 -> Divide7/1
  Divide7/1 -> Add2/3
  Trigonometric Function3/1 -> Divide2/3, Divide5/3, Divide3/3
  Trigonometric Function5/1 -> Divide4/1, Divide5/2
  Trigonometric Function4/1 -> Divide4/2, Divide6/2
  Trigonometric Function2/1 -> Divide2/1, Divide5/1
  Trigonometric Function/1 -> Divide2/2, Divide6/1
  Demux1/3 -> Divide7/2
  Demux1/2 -> Divide1/2
  Demux2/1 -> Trigonometric Function5/1, Trigonometric Function/1
  Demux2/2 -> Trigonometric Function1/1, Trigonometric Function2/1
  Demux2/3 -> Trigonometric Function4/1, Trigonometric Function3/1

== system NavigationObserver_4/Navigation Observer/EKF/K[k] (navigation)/Jacobian F/f_(x_est_[k],u_[k])+delta_ve/f(x_est_[k],u_[k])/f(vh_est_[k];u) ==
  note: phi [rad]
  note: theta [rad]
  note: az [ft/sec2]
  note: ay [ft/sec2]
  note: ax [ft/sec2]
  Accelerometer Meas : Inport
  "phi, theta, psi" : Inport  Port=2
  Add1 : Sum  Inputs=+--
  Demux1 : Demux  Outputs=3
  Demux2 : Demux  Outputs=3
  Divide1 : Product  Inputs=***
  Divide2 : Product  Inputs=**
  Divide3 : Product  Inputs=***
  Sum : Sum  Inputs=|+-  SampleTime=dt
  Terminator2 : Terminator
  Trigonometric Function : Trigonometry
  Trigonometric Function1 : Trigonometry  Operator=cos
  Trigonometric Function2 : Trigonometry
  Trigonometric Function4 : Trigonometry  Operator=cos
  Trigonometric Function5 : Trigonometry  Operator=cos
  gravity : Constant  Value=g
  f(vh_est_[k];u) : Outport
  wires:
  gravity/1 -> Sum/2
  Sum/1 -> f(vh_est_[k];u)/1
  Add1/1 -> Sum/1
  Demux2/3 -> Terminator2/1
  "phi, theta, psi"/1 -> Demux2/1
  Accelerometer Meas/1 -> Demux1/1
  Demux1/1 -> Divide2/1
  Trigonometric Function/1 -> Divide2/2
  Trigonometric Function1/1 -> Divide3/1
  Trigonometric Function2/1 -> Divide3/2
  Demux1/2 -> Divide3/3
  Divide3/1 -> Add1/2
  Divide2/1 -> Add1/1
  Trigonometric Function4/1 -> Divide1/1
  Trigonometric Function5/1 -> Divide1/2
  Demux1/3 -> Divide1/3
  Divide1/1 -> Add1/3
  Demux2/2 -> Trigonometric Function/1, Trigonometric Function1/1, Trigonometric Function5/1
  Demux2/1 -> Trigonometric Function2/1, Trigonometric Function4/1

== system NavigationObserver_4/Navigation Observer/EKF/K[k] (navigation)/Jacobian F/f_(x_est_[k],u_[k])+delta_ve/f(x_est_[k],u_[k])/f(vn_est_[k];u) ==
  note: psi [rad]
  note: phi [rad]
  note: theta [rad]
  note: az [ft/sec2]
  note: ay [ft/sec2]
  note: ax [ft/sec2]
  Accelerometer Meas : Inport
  "phi, theta, psi" : Inport  Port=2
  Add1 : Sum  Inputs=-+
  Add2 : Sum  Inputs=+++
  Add3 : Sum
  Demux1 : Demux  Outputs=3
  Demux2 : Demux  Outputs=3
  Divide{1,4,6..7} (4 alike) : Product  Inputs=**
  Divide2 : Product  Inputs=***
  Divide3 : Product  Inputs=***
  Divide5 : Product  Inputs=***
  Trigonometric Function : Trigonometry
  Trigonometric Function1 : Trigonometry  Operator=cos
  Trigonometric Function2 : Trigonometry
  Trigonometric Function3 : Trigonometry
  Trigonometric Function4 : Trigonometry  Operator=cos
  Trigonometric Function5 : Trigonometry  Operator=cos
  f(vn_est_[k];u) : Outport
  wires:
  Accelerometer Meas/1 -> Demux1/1
  Demux1/1 -> Divide3/1
  Demux1/2 -> Divide1/2
  Demux1/3 -> Divide7/2
  Add2/1 -> f(vn_est_[k];u)/1
  Demux2/2 -> Trigonometric Function1/1, Trigonometric Function2/1
  Demux2/1 -> Trigonometric Function5/1, Trigonometric Function/1
  Demux2/3 -> Trigonometric Function4/1, Trigonometric Function3/1
  Trigonometric Function1/1 -> Divide3/2
  Trigonometric Function4/1 -> Divide3/3, Divide2/3, Divide5/3
  Add1/1 -> Divide1/1
  Divide4/1 -> Add1/1
  Divide2/1 -> Add1/2
  Trigonometric Function5/1 -> Divide4/1, Divide5/2
  Trigonometric Function3/1 -> Divide4/2, Divide6/2
  Trigonometric Function2/1 -> Divide2/1, Divide5/1
  Trigonometric Function/1 -> Divide2/2, Divide6/1
  Divide3/1 -> Add2/1
  Divide1/1 -> Add2/2
  Divide6/1 -> Add3/1
  Divide5/1 -> Add3/2
  Add3/1 -> Divide7/1
  Divide7/1 -> Add2/3
  "phi, theta, psi"/1 -> Demux2/1

== system NavigationObserver_4/Navigation Observer/EKF/K[k] (navigation)/Jacobian F/f_(x_est_[k],u_[k])+delta_ve/f(x_est_[k],u_[k])/f_pe(x_est_[k],u[k]) ==
  Gain : Gain
  f_pe(x_est_[k],u[k]) : Outport
  wires:
  Gain/1 -> f_pe(x_est_[k],u[k])/1
  [ve_o] -> Gain/1

== system NavigationObserver_4/Navigation Observer/EKF/K[k] (navigation)/Jacobian F/f_(x_est_[k],u_[k])+delta_ve/f(x_est_[k],u_[k])/f_ph(x_est_[k],u[k]) ==
  Gain : Gain
  f_ph(x_est_[k],u[k]) : Outport
  wires:
  Gain/1 -> f_ph(x_est_[k],u[k])/1
  [vh_o] -> Gain/1

== system NavigationObserver_4/Navigation Observer/EKF/K[k] (navigation)/Jacobian F/f_(x_est_[k],u_[k])+delta_ve/f(x_est_[k],u_[k])/f_pn(x_est_[k],u[k]) ==
  Gain : Gain
  f_pn(x_est_[k],u[k]) : Outport
  wires:
  Gain/1 -> f_pn(x_est_[k],u[k])/1
  [vn_o] -> Gain/1

== system NavigationObserver_4/Navigation Observer/EKF/K[k] (navigation)/Jacobian F/f_(x_est_[k],u_[k])+delta_vh/f(x_est_[k],u_[k])/f(ve_est_[k];u) ==
  note: psi [rad]
  note: phi [rad]
  note: theta [rad]
  note: az [ft/sec2]
  note: ay [ft/sec2]
  note: ax [ft/sec2]
  Accelerometer Meas : Inport
  "phi, theta, psi" : Inport  Port=2
  Add1 : Sum
  Add2 : Sum  Inputs=+++
  Add3 : Sum  Inputs=-+
  Demux1 : Demux  Outputs=3
  Demux2 : Demux  Outputs=3
  Divide{1,4,6..7} (4 alike) : Product  Inputs=**
  Divide2 : Product  Inputs=***
  Divide3 : Product  Inputs=***
  Divide5 : Product  Inputs=***
  Trigonometric Function : Trigonometry
  Trigonometric Function1 : Trigonometry  Operator=cos
  Trigonometric Function2 : Trigonometry
  Trigonometric Function3 : Trigonometry
  Trigonometric Function4 : Trigonometry  Operator=cos
  Trigonometric Function5 : Trigonometry  Operator=cos
  f(ve_est_[k];u) : Outport
  wires:
  "phi, theta, psi"/1 -> Demux2/1
  Accelerometer Meas/1 -> Demux1/1
  Add2/1 -> f(ve_est_[k];u)/1
  Demux1/1 -> Divide3/1
  Trigonometric Function1/1 -> Divide3/2
  Add1/1 -> Divide1/1
  Divide4/1 -> Add1/1
  Divide2/1 -> Add1/2
  Divide3/1 -> Add2/1
  Divide1/1 -> Add2/2
  Divide6/1 -> Add3/1
  Divide5/1 -> Add3/2
  Add3/1 -> Divide7/1
  Divide7/1 -> Add2/3
  Trigonometric Function3/1 -> Divide2/3, Divide5/3, Divide3/3
  Trigonometric Function5/1 -> Divide4/1, Divide5/2
  Trigonometric Function4/1 -> Divide4/2, Divide6/2
  Trigonometric Function2/1 -> Divide2/1, Divide5/1
  Trigonometric Function/1 -> Divide2/2, Divide6/1
  Demux1/3 -> Divide7/2
  Demux1/2 -> Divide1/2
  Demux2/1 -> Trigonometric Function5/1, Trigonometric Function/1
  Demux2/2 -> Trigonometric Function1/1, Trigonometric Function2/1
  Demux2/3 -> Trigonometric Function4/1, Trigonometric Function3/1

== system NavigationObserver_4/Navigation Observer/EKF/K[k] (navigation)/Jacobian F/f_(x_est_[k],u_[k])+delta_vh/f(x_est_[k],u_[k])/f(vh_est_[k];u) ==
  note: phi [rad]
  note: theta [rad]
  note: az [ft/sec2]
  note: ay [ft/sec2]
  note: ax [ft/sec2]
  Accelerometer Meas : Inport
  "phi, theta, psi" : Inport  Port=2
  Add1 : Sum  Inputs=+--
  Demux1 : Demux  Outputs=3
  Demux2 : Demux  Outputs=3
  Divide1 : Product  Inputs=***
  Divide2 : Product  Inputs=**
  Divide3 : Product  Inputs=***
  Sum : Sum  Inputs=|+-  SampleTime=dt
  Terminator2 : Terminator
  Trigonometric Function : Trigonometry
  Trigonometric Function1 : Trigonometry  Operator=cos
  Trigonometric Function2 : Trigonometry
  Trigonometric Function4 : Trigonometry  Operator=cos
  Trigonometric Function5 : Trigonometry  Operator=cos
  gravity : Constant  Value=g
  f(vh_est_[k];u) : Outport
  wires:
  gravity/1 -> Sum/2
  Sum/1 -> f(vh_est_[k];u)/1
  Add1/1 -> Sum/1
  Demux2/3 -> Terminator2/1
  "phi, theta, psi"/1 -> Demux2/1
  Accelerometer Meas/1 -> Demux1/1
  Demux1/1 -> Divide2/1
  Trigonometric Function/1 -> Divide2/2
  Trigonometric Function1/1 -> Divide3/1
  Trigonometric Function2/1 -> Divide3/2
  Demux1/2 -> Divide3/3
  Divide3/1 -> Add1/2
  Divide2/1 -> Add1/1
  Trigonometric Function4/1 -> Divide1/1
  Trigonometric Function5/1 -> Divide1/2
  Demux1/3 -> Divide1/3
  Divide1/1 -> Add1/3
  Demux2/2 -> Trigonometric Function/1, Trigonometric Function1/1, Trigonometric Function5/1
  Demux2/1 -> Trigonometric Function2/1, Trigonometric Function4/1

== system NavigationObserver_4/Navigation Observer/EKF/K[k] (navigation)/Jacobian F/f_(x_est_[k],u_[k])+delta_vh/f(x_est_[k],u_[k])/f(vn_est_[k];u) ==
  note: psi [rad]
  note: phi [rad]
  note: theta [rad]
  note: az [ft/sec2]
  note: ay [ft/sec2]
  note: ax [ft/sec2]
  Accelerometer Meas : Inport
  "phi, theta, psi" : Inport  Port=2
  Add1 : Sum  Inputs=-+
  Add2 : Sum  Inputs=+++
  Add3 : Sum
  Demux1 : Demux  Outputs=3
  Demux2 : Demux  Outputs=3
  Divide{1,4,6..7} (4 alike) : Product  Inputs=**
  Divide2 : Product  Inputs=***
  Divide3 : Product  Inputs=***
  Divide5 : Product  Inputs=***
  Trigonometric Function : Trigonometry
  Trigonometric Function1 : Trigonometry  Operator=cos
  Trigonometric Function2 : Trigonometry
  Trigonometric Function3 : Trigonometry
  Trigonometric Function4 : Trigonometry  Operator=cos
  Trigonometric Function5 : Trigonometry  Operator=cos
  f(vn_est_[k];u) : Outport
  wires:
  Accelerometer Meas/1 -> Demux1/1
  Demux1/1 -> Divide3/1
  Demux1/2 -> Divide1/2
  Demux1/3 -> Divide7/2
  Add2/1 -> f(vn_est_[k];u)/1
  Demux2/2 -> Trigonometric Function1/1, Trigonometric Function2/1
  Demux2/1 -> Trigonometric Function5/1, Trigonometric Function/1
  Demux2/3 -> Trigonometric Function4/1, Trigonometric Function3/1
  Trigonometric Function1/1 -> Divide3/2
  Trigonometric Function4/1 -> Divide3/3, Divide2/3, Divide5/3
  Add1/1 -> Divide1/1
  Divide4/1 -> Add1/1
  Divide2/1 -> Add1/2
  Trigonometric Function5/1 -> Divide4/1, Divide5/2
  Trigonometric Function3/1 -> Divide4/2, Divide6/2
  Trigonometric Function2/1 -> Divide2/1, Divide5/1
  Trigonometric Function/1 -> Divide2/2, Divide6/1
  Divide3/1 -> Add2/1
  Divide1/1 -> Add2/2
  Divide6/1 -> Add3/1
  Divide5/1 -> Add3/2
  Add3/1 -> Divide7/1
  Divide7/1 -> Add2/3
  "phi, theta, psi"/1 -> Demux2/1

== system NavigationObserver_4/Navigation Observer/EKF/K[k] (navigation)/Jacobian F/f_(x_est_[k],u_[k])+delta_vh/f(x_est_[k],u_[k])/f_pe(x_est_[k],u[k]) ==
  Gain : Gain
  f_pe(x_est_[k],u[k]) : Outport
  wires:
  Gain/1 -> f_pe(x_est_[k],u[k])/1
  [ve_o] -> Gain/1

== system NavigationObserver_4/Navigation Observer/EKF/K[k] (navigation)/Jacobian F/f_(x_est_[k],u_[k])+delta_vh/f(x_est_[k],u_[k])/f_ph(x_est_[k],u[k]) ==
  Gain : Gain
  f_ph(x_est_[k],u[k]) : Outport
  wires:
  Gain/1 -> f_ph(x_est_[k],u[k])/1
  [vh_o] -> Gain/1

== system NavigationObserver_4/Navigation Observer/EKF/K[k] (navigation)/Jacobian F/f_(x_est_[k],u_[k])+delta_vh/f(x_est_[k],u_[k])/f_pn(x_est_[k],u[k]) ==
  Gain : Gain
  f_pn(x_est_[k],u[k]) : Outport
  wires:
  Gain/1 -> f_pn(x_est_[k],u[k])/1
  [vn_o] -> Gain/1

== system NavigationObserver_4/Navigation Observer/EKF/K[k] (navigation)/Jacobian F/f_(x_est_[k],u_[k])+delta_vn/f(x_est_[k],u_[k])/f(ve_est_[k];u) ==
  note: psi [rad]
  note: phi [rad]
  note: theta [rad]
  note: az [ft/sec2]
  note: ay [ft/sec2]
  note: ax [ft/sec2]
  Accelerometer Meas : Inport
  "phi, theta, psi" : Inport  Port=2
  Add1 : Sum
  Add2 : Sum  Inputs=+++
  Add3 : Sum  Inputs=-+
  Demux1 : Demux  Outputs=3
  Demux2 : Demux  Outputs=3
  Divide{1,4,6..7} (4 alike) : Product  Inputs=**
  Divide2 : Product  Inputs=***
  Divide3 : Product  Inputs=***
  Divide5 : Product  Inputs=***
  Trigonometric Function : Trigonometry
  Trigonometric Function1 : Trigonometry  Operator=cos
  Trigonometric Function2 : Trigonometry
  Trigonometric Function3 : Trigonometry
  Trigonometric Function4 : Trigonometry  Operator=cos
  Trigonometric Function5 : Trigonometry  Operator=cos
  f(ve_est_[k];u) : Outport
  wires:
  "phi, theta, psi"/1 -> Demux2/1
  Accelerometer Meas/1 -> Demux1/1
  Add2/1 -> f(ve_est_[k];u)/1
  Demux1/1 -> Divide3/1
  Trigonometric Function1/1 -> Divide3/2
  Add1/1 -> Divide1/1
  Divide4/1 -> Add1/1
  Divide2/1 -> Add1/2
  Divide3/1 -> Add2/1
  Divide1/1 -> Add2/2
  Divide6/1 -> Add3/1
  Divide5/1 -> Add3/2
  Add3/1 -> Divide7/1
  Divide7/1 -> Add2/3
  Trigonometric Function3/1 -> Divide2/3, Divide5/3, Divide3/3
  Trigonometric Function5/1 -> Divide4/1, Divide5/2
  Trigonometric Function4/1 -> Divide4/2, Divide6/2
  Trigonometric Function2/1 -> Divide2/1, Divide5/1
  Trigonometric Function/1 -> Divide2/2, Divide6/1
  Demux1/3 -> Divide7/2
  Demux1/2 -> Divide1/2
  Demux2/1 -> Trigonometric Function5/1, Trigonometric Function/1
  Demux2/2 -> Trigonometric Function1/1, Trigonometric Function2/1
  Demux2/3 -> Trigonometric Function4/1, Trigonometric Function3/1

== system NavigationObserver_4/Navigation Observer/EKF/K[k] (navigation)/Jacobian F/f_(x_est_[k],u_[k])+delta_vn/f(x_est_[k],u_[k])/f(vh_est_[k];u) ==
  note: phi [rad]
  note: theta [rad]
  note: az [ft/sec2]
  note: ay [ft/sec2]
  note: ax [ft/sec2]
  Accelerometer Meas : Inport
  "phi, theta, psi" : Inport  Port=2
  Add1 : Sum  Inputs=+--
  Demux1 : Demux  Outputs=3
  Demux2 : Demux  Outputs=3
  Divide1 : Product  Inputs=***
  Divide2 : Product  Inputs=**
  Divide3 : Product  Inputs=***
  Sum : Sum  Inputs=|+-  SampleTime=dt
  Terminator2 : Terminator
  Trigonometric Function : Trigonometry
  Trigonometric Function1 : Trigonometry  Operator=cos
  Trigonometric Function2 : Trigonometry
  Trigonometric Function4 : Trigonometry  Operator=cos
  Trigonometric Function5 : Trigonometry  Operator=cos
  gravity : Constant  Value=g
  f(vh_est_[k];u) : Outport
  wires:
  gravity/1 -> Sum/2
  Sum/1 -> f(vh_est_[k];u)/1
  Add1/1 -> Sum/1
  Demux2/3 -> Terminator2/1
  "phi, theta, psi"/1 -> Demux2/1
  Accelerometer Meas/1 -> Demux1/1
  Demux1/1 -> Divide2/1
  Trigonometric Function/1 -> Divide2/2
  Trigonometric Function1/1 -> Divide3/1
  Trigonometric Function2/1 -> Divide3/2
  Demux1/2 -> Divide3/3
  Divide3/1 -> Add1/2
  Divide2/1 -> Add1/1
  Trigonometric Function4/1 -> Divide1/1
  Trigonometric Function5/1 -> Divide1/2
  Demux1/3 -> Divide1/3
  Divide1/1 -> Add1/3
  Demux2/2 -> Trigonometric Function/1, Trigonometric Function1/1, Trigonometric Function5/1
  Demux2/1 -> Trigonometric Function2/1, Trigonometric Function4/1

== system NavigationObserver_4/Navigation Observer/EKF/K[k] (navigation)/Jacobian F/f_(x_est_[k],u_[k])+delta_vn/f(x_est_[k],u_[k])/f(vn_est_[k];u) ==
  note: psi [rad]
  note: phi [rad]
  note: theta [rad]
  note: az [ft/sec2]
  note: ay [ft/sec2]
  note: ax [ft/sec2]
  Accelerometer Meas : Inport
  "phi, theta, psi" : Inport  Port=2
  Add1 : Sum  Inputs=-+
  Add2 : Sum  Inputs=+++
  Add3 : Sum
  Demux1 : Demux  Outputs=3
  Demux2 : Demux  Outputs=3
  Divide{1,4,6..7} (4 alike) : Product  Inputs=**
  Divide2 : Product  Inputs=***
  Divide3 : Product  Inputs=***
  Divide5 : Product  Inputs=***
  Trigonometric Function : Trigonometry
  Trigonometric Function1 : Trigonometry  Operator=cos
  Trigonometric Function2 : Trigonometry
  Trigonometric Function3 : Trigonometry
  Trigonometric Function4 : Trigonometry  Operator=cos
  Trigonometric Function5 : Trigonometry  Operator=cos
  f(vn_est_[k];u) : Outport
  wires:
  Accelerometer Meas/1 -> Demux1/1
  Demux1/1 -> Divide3/1
  Demux1/2 -> Divide1/2
  Demux1/3 -> Divide7/2
  Add2/1 -> f(vn_est_[k];u)/1
  Demux2/2 -> Trigonometric Function1/1, Trigonometric Function2/1
  Demux2/1 -> Trigonometric Function5/1, Trigonometric Function/1
  Demux2/3 -> Trigonometric Function4/1, Trigonometric Function3/1
  Trigonometric Function1/1 -> Divide3/2
  Trigonometric Function4/1 -> Divide3/3, Divide2/3, Divide5/3
  Add1/1 -> Divide1/1
  Divide4/1 -> Add1/1
  Divide2/1 -> Add1/2
  Trigonometric Function5/1 -> Divide4/1, Divide5/2
  Trigonometric Function3/1 -> Divide4/2, Divide6/2
  Trigonometric Function2/1 -> Divide2/1, Divide5/1
  Trigonometric Function/1 -> Divide2/2, Divide6/1
  Divide3/1 -> Add2/1
  Divide1/1 -> Add2/2
  Divide6/1 -> Add3/1
  Divide5/1 -> Add3/2
  Add3/1 -> Divide7/1
  Divide7/1 -> Add2/3
  "phi, theta, psi"/1 -> Demux2/1

== system NavigationObserver_4/Navigation Observer/EKF/K[k] (navigation)/Jacobian F/f_(x_est_[k],u_[k])+delta_vn/f(x_est_[k],u_[k])/f_pe(x_est_[k],u[k]) ==
  Gain : Gain
  f_pe(x_est_[k],u[k]) : Outport
  wires:
  Gain/1 -> f_pe(x_est_[k],u[k])/1
  [ve_o] -> Gain/1

== system NavigationObserver_4/Navigation Observer/EKF/K[k] (navigation)/Jacobian F/f_(x_est_[k],u_[k])+delta_vn/f(x_est_[k],u_[k])/f_ph(x_est_[k],u[k]) ==
  Gain : Gain
  f_ph(x_est_[k],u[k]) : Outport
  wires:
  Gain/1 -> f_ph(x_est_[k],u[k])/1
  [vh_o] -> Gain/1

== system NavigationObserver_4/Navigation Observer/EKF/K[k] (navigation)/Jacobian F/f_(x_est_[k],u_[k])+delta_vn/f(x_est_[k],u_[k])/f_pn(x_est_[k],u[k]) ==
  Gain : Gain
  f_pn(x_est_[k],u[k]) : Outport
  wires:
  Gain/1 -> f_pn(x_est_[k],u[k])/1
  [vn_o] -> Gain/1

== matlab function Navigation Observer/EKF/K[k] (navigation)/K_[k]/Inverse ==
  data: u input double; y output double
function y = fcn(u)
%#codegen

y = u^-1;

== matlab function Navigation Observer/EKF/K[k] (navigation)/K_[k]/Transpose ==
  data: u input double; HT_k output double
function HT_k = fcn(u)
%#codegen

HT_k = u';

== matlab function Navigation Observer/EKF/K[k] (navigation)/Transpose ==
  data: u input double; FT_k_1 output double
function FT_k_1 = fcn(u)
%#codegen

FT_k_1 = u';

== matlab function Navigation Observer/GPS to Local/Convert Lat//Lon//Alt to Flat Earth ==
  data: wpts input double; Height output double; alt input double; lat input double; lon input double; North output double; East output double
function [Height, North, East] = lla_to_fe(wpts, alt, lat, lon)

% Convert the given LLA coordinates to Flat Earth coordinates.
%
% ref_alt - meters ASML
% ref_lat - deg.
% ref_lon - deg.
%
% Height, North, East are in feet

Height = (alt - wpts.ref_alt)*(1/0.3048);
North  = (lat - wpts.ref_lat)*(wpts.fact_lat);
East   = (lon - wpts.ref_lon)*(wpts.fact_lon);

== matlab function Navigation Observer/Local Position to GPS Position/Convert Local Coordinates to LLA ==
  data: n input double; Latitude output double; e input double; h input double; Longitude output double; Altitude output double; wpts input double
function [Latitude, Longitude, Altitude] = local_to_lla(n, e, h, wpts)


Latitude  = n/wpts.fact_lat + wpts.ref_lat;
Longitude = e/wpts.fact_lon + wpts.ref_lon;
Altitude  = h*0.3048        + wpts.ref_alt;
